simulink model "WMR_ROS_MATMPC_SIMULINK"  (R2022b)
settings: Solver=FixedStepAuto  StartTime=0.0  StopTime=20  FixedStep=0.001  RelTol=1e-3
values from neighbouring files (symbols this model uses):
  lb = 0    [Initialization_Simulink.m]
  lbu = -inf(nu,1)    [InitData.m]    (also in Initialization_Simulink.m = repmat(lbu,1,N))
  lbx = 0    [Initialization_Simulink.m]
  N = settings.N    [InitData.m]    (also in InitMemory.m; Initialization_Simulink.m = 160; Simulation.m = 10)
  para = repmat(para0,1,N+1)    [InitData.m]    (also in Initialization_Simulink.m)
  Ts = settings.Ts_st    [Initialization_Simulink.m]    (also in Simulation.m)
  ub = 0    [Initialization_Simulink.m]
  ubu = inf(nu,1)    [InitData.m]    (also in Initialization_Simulink.m = repmat(ubu,1,N))
  ubx = 0    [Initialization_Simulink.m]
  W = repmat([1 1 0.001 1 1 5 10]',1,N)    [Initialization_Simulink.m]
  WN = [100 100 0.001 10 10]'    [Initialization_Simulink.m]
  yref = 1    [run_experiment_gazebo.m]    (also in run_experiment_move_base.m; run_experiment_simulink.m = 2)
  z0 = 0    [Initialization_Simulink.m]
  zref = 2    [run_experiment_gazebo.m]    (also in run_experiment_move_base.m = 4; run_experiment_simulink.m = 4)
undefined symbols (not defined in the file or in its folder): Angular, Linear, opt, settings, X, X_SL_Info, Y, Y_SL_Info
libraries: robotlib x5, robotgazebolib x1, robotcorelib x1
settings Model: Creator=chen  LastModifiedBy=davidedl
settings SolverCC: AlgebraicLoopSolver=TrustRegion
settings DataIOCC: ReturnWorkspaceOutputs=off
settings OptimizationCC: EnhancedBackFolding=on  PassReuseOutputArgsAs=Individual arguments  ZeroExternalMemoryAtStartup=off  ZeroInternalMemoryAtStartup=off  MaxStackSize=64  OptimizeBlockOrder=speed  DifferentSizesBufferReuse=on  OptimizationCustomize=off  EfficientTunableParamExpr=on
settings DebuggingCC: ParameterTunabilityLossMsg=error  UnconnectedInputMsg=warning  UnconnectedOutputMsg=warning  UnconnectedLineMsg=warning  SFMachineParentedDataDiag=warning  ArithmeticOperatorsInVariantConditions=warning
settings HardwareCC: ProdBitPerPointer=32  ProdBitPerSizeT=32  ProdBitPerPtrDiffT=32  ProdLargestAtomicFloat=None  ProdIntDivRoundTo=Undefined  ProdEndianess=Unspecified  ProdWordSize=32  ProdHWDeviceType=Generic->Unspecified (assume 32-bit Generic)  UseEmbeddedCoderFeatures=off
settings ModelReferenceCC: EnableRefExpFcnMdlSchedulingChecks=on
settings SFSimCC: SimUseLocalCustomCode=off  MATLABDynamicMemAlloc=off  CustomCodeUndefinedFunction=UseInterfaceOnly
settings RTWCC: Description=Embedded Coder  SystemTargetFile=ert.tlc  HardwareBoard=Robot Operating System (ROS)  TLCOptions="-aInlineSetEventsForThisBaseRateFcn=TLC_FALSE -aSuppressMultiTaskScheduler=TLC_FALSE  -aRateBasedStepFcn=0"  TemplateMakefile=ert_default_tmf  RTWUseLocalCustomCode=off  Toolchain=Catkin  TargetLang=C++  CheckMdlBeforeBuild=Error
settings CodeAppCC: ForceParamTrailComments=on  IgnoreCustomStorageClasses=off  OperatorAnnotations=on  SimulinkDataObjDesc=on  SFDataObjDesc=on  InsertBlockDesc=on
settings ERTTargetCC: SupportNonInlinedSFcns=on

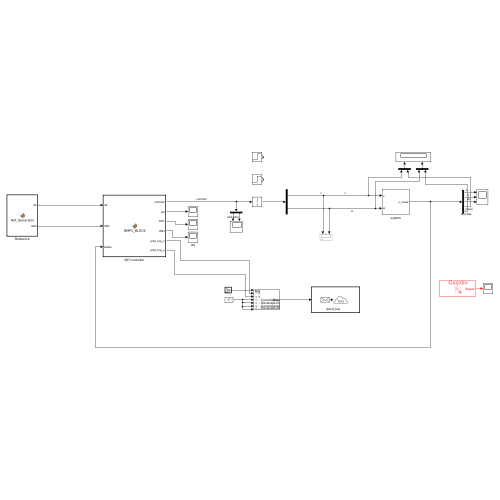
[thumbnail: Simulink's stored preview of the top-level diagram]
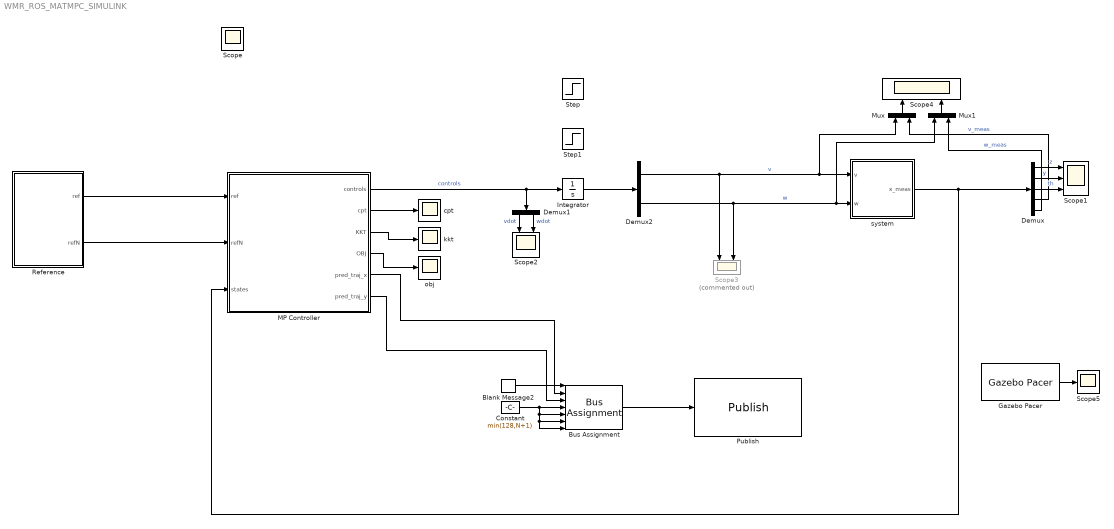
== system WMR_ROS_MATMPC_SIMULINK ==
  Blank Message2 : robotlib/Blank Message  messageClass=Message  entityType=wheelchair_iaslab_control/matArray  messageType=wheelchair_iaslab_control/matArray  SampleTime=-1  legacyBusStruct=off
  Bus Assignment : BusAssignment  AssignedSignals=X,Y,X_SL_Info.CurrentLength,X_SL_Info.ReceivedLength,Y_SL_Info.CurrentLength,Y_SL_Info.ReceivedLength
  Constant : Constant  Value=min(128,N+1)  OutDataTypeStr=uint32
  Demux : Demux  Outputs=5
  Demux1 : Demux  Outputs=2
  Demux2 : Demux  Outputs=2
  Gazebo Pacer : robotgazebolib/Gazebo Pacer  ResetBehavior=Reset Gazebo simulation time and scene  SampleTime=0.001
  Integrator : Integrator  InitialCondition=[0,0]
  MP Controller : MATLAB Function  TreatAsAtomicUnit=on  SystemSampleTime=Ts
  Mux : Mux  Inputs=2
  Mux1 : Mux  Inputs=2
  Publish : robotlib/Publish  topicSource=Specify your own  topic=/pred_traj  messageType=wheelchair_iaslab_control/matArray  legacyBusStruct=off  messageQueueLength=1
      settings: LibrarySourceBlock=roslib/ROS/Publish
  Reference : MATLAB Function  TreatAsAtomicUnit=on
  Scope1 : Scope  NumInputPorts=3
  Scope2 : Scope  NumInputPorts=2
  Scope3 : Scope  Commented=on  NumInputPorts=2
  Scope4 : Scope  NumInputPorts=2
  Scope5 : Scope
  Step : Step  Time=9  After=0  SampleTime=0
  Step1 : Step  Time=9  After=0  SampleTime=0
  cpt : Scope
  kkt : Scope
  obj : Scope
  system : Subsystem
  Scope : Scope
  wires:
  MP Controller/1(controls) -> Integrator/1, Demux1/1  "controls"
  MP Controller/2(cpt) -> cpt/1
  MP Controller/4(OBJ) -> obj/1
  MP Controller/3(KKT) -> kkt/1
  Reference/1(ref) -> MP Controller/1(ref)
  Reference/2(refN) -> MP Controller/2(refN)
  Integrator/1 -> Demux2/1
  Demux2/1 -> Scope3/1, Mux/1, system/1(v)  "v"
  Demux2/2 -> Mux1/1, system/2(w), Scope3/2  "w"
  Demux/3 -> Scope1/3  "th"
  Demux/1 -> Scope1/1  "z"
  Demux/2 -> Scope1/2  "y"
  Demux/5 -> Mux1/2  "w_meas"
  Demux/4 -> Mux/2  "v_meas"
  Demux1/1 -> Scope2/1  "vdot"
  Demux1/2 -> Scope2/2  "wdot"
  system/1(x_meas) -> MP Controller/3(states), Demux/1
  Mux/1 -> Scope4/1
  Mux1/1 -> Scope4/2
  Blank Message2/1 -> Bus Assignment/1
  Bus Assignment/1 -> Publish/1
  MP Controller/5(pred_traj_x) -> Bus Assignment/2
  MP Controller/6(pred_traj_y) -> Bus Assignment/3
  Gazebo Pacer/1 -> Scope5/1
  Constant/1 -> Bus Assignment/7, Bus Assignment/6, Bus Assignment/5, Bus Assignment/4

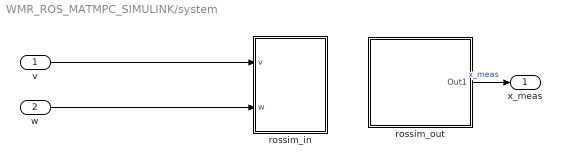
== system WMR_ROS_MATMPC_SIMULINK/system ==
  v : Inport
  w : Inport  Port=2
  rossim_in : Subsystem
  rossim_out : Subsystem
  x_meas : Outport
  wires:
  w/1 -> rossim_in/2(w)
  v/1 -> rossim_in/1(v)
  rossim_out/1(Out1) -> x_meas/1  "x_meas"

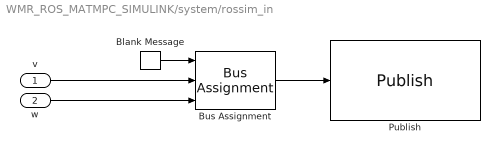
== system WMR_ROS_MATMPC_SIMULINK/system/rossim_in ==
  v : Inport
  w : Inport  Port=2
  Blank Message : robotlib/Blank Message  messageClass=Message  entityType=geometry_msgs/Twist  messageType=geometry_msgs/Twist  SampleTime=-1  legacyBusStruct=off
  Bus Assignment : BusAssignment  AssignedSignals=Linear.X,Angular.Z
  Publish : robotlib/Publish  topicSource=Specify your own  topic=/wcias_controller/cmd_vel  messageType=geometry_msgs/Twist  legacyBusStruct=off  messageQueueLength=1
      settings: LibrarySourceBlock=roslib/ROS/Publish
  wires:
  Blank Message/1 -> Bus Assignment/1
  Bus Assignment/1 -> Publish/1
  w/1 -> Bus Assignment/3
  v/1 -> Bus Assignment/2

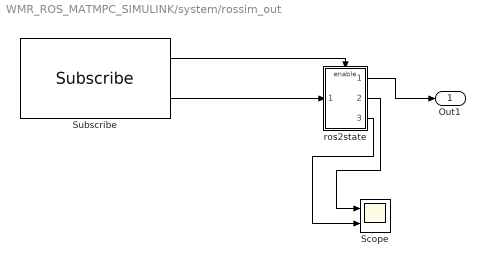
== system WMR_ROS_MATMPC_SIMULINK/system/rossim_out ==
  Scope : Scope  NumInputPorts=2
  Subscribe : robotlib/Subscribe  topicSource=Specify your own  topic=/wcias_controller/odom  messageType=nav_msgs/Odometry  SampleTime=0.001  legacyBusStruct=off  messageQueueLength=1
      settings: LibrarySourceBlock=roslib/ROS/Subscribe
  ros2state : Subsystem
  Out1 : Outport
  wires:
  Subscribe/1 -> ros2state/Enable
  Subscribe/2 -> ros2state/1(In1)
  ros2state/1(Out1) -> Out1/1
  ros2state/2(Out2) -> Scope/1
  ros2state/3(Out3) -> Scope/2

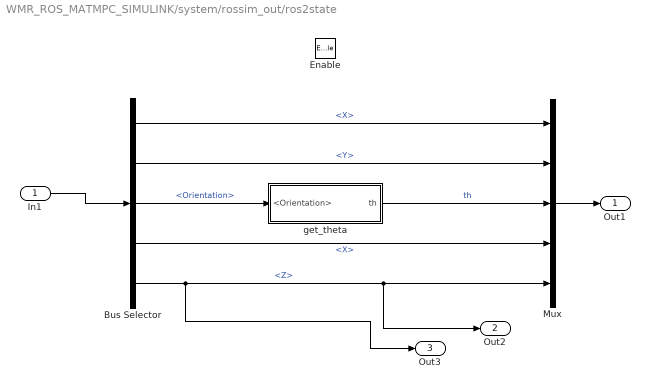
== system WMR_ROS_MATMPC_SIMULINK/system/rossim_out/ros2state ==
  In1 : Inport
  Enable : EnablePort  StatesWhenEnabling=reset
  Bus Selector : BusSelector  DialogController=Simulink.DDGSource_BusSelector  OutputSignals=Pose.Pose.Position.X,Pose.Pose.Position.Y,Pose.Pose.Orientation,Twist.Twist.Linear.X,Twist.Twist.Angular.Z
  Mux : Mux  Inputs=5
  get_theta : Subsystem
  Out1 : Outport
  Out2 : Outport  Port=2
  Out3 : Outport  Port=3
  wires:
  Bus Selector/5 -> Mux/5, Out2/1, Out3/1  "<Z>"
  Bus Selector/1 -> Mux/1  "<X>"
  In1/1 -> Bus Selector/1
  get_theta/1(th) -> Mux/3  "th"
  Bus Selector/2 -> Mux/2  "<Y>"
  Bus Selector/3 -> get_theta/1(<Orientation>)  "<Orientation>"
  Bus Selector/4 -> Mux/4  "<X>"
  Mux/1 -> Out1/1

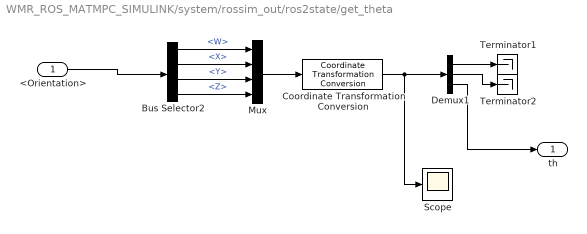
== system WMR_ROS_MATMPC_SIMULINK/system/rossim_out/ros2state/get_theta ==
  <Orientation> : Inport
  Bus Selector2 : BusSelector  DialogController=Simulink.DDGSource_BusSelector  OutputSignals=W,X,Y,Z
  Coordinate Transformation Conversion : robotcorelib/Coordinate Transformation Conversion  InputRepresentation=Quaternion  InputEulerSequence=ZYX  ShowTrVecInputPort=on  OutputRepresentation=Euler Angles  OutputEulerSequence=XYZ  ShowTrVecOutputPort=on  SimulateUsing=Interpreted execution
      settings: LibrarySourceBlock=roslib/Utilities/Coordinate Transformation Conversion
  Demux1 : Demux  Outputs=3
  Mux : Mux
  Scope : Scope
  Terminator1 : Terminator
  Terminator2 : Terminator
  th : Outport
  wires:
  Bus Selector2/3 -> Mux/3  "<Y>"
  Demux1/1 -> Terminator1/1
  Bus Selector2/4 -> Mux/4  "<Z>"
  Bus Selector2/1 -> Mux/1  "<W>"
  Coordinate Transformation Conversion/1 -> Scope/1, Demux1/1
  <Orientation>/1 -> Bus Selector2/1
  Demux1/2 -> Terminator2/1
  Bus Selector2/2 -> Mux/2  "<X>"
  Mux/1 -> Coordinate Transformation Conversion/1
  Demux1/3 -> th/1

== matlab function WMR_ROS_MATMPC_SIMULINK/Reference ==
  data: ref output; settings parameter; refN output; zref parameter; yref parameter
function [ref,refN] = Ref_Generator(settings, zref, yref)

    ref = repmat([zref,yref,0,0,0,0,0]',1,settings.N);
    refN = [zref,yref,0,0,0]';

end

== matlab function WMR_ROS_MATMPC_SIMULINK/MP Controller ==
  settings: updateMethod=DISCRETE  sampleTime=1/50
  data: settings parameter; opt parameter; lb parameter; ub parameter; lbx parameter; ubx parameter; lbu parameter; ubu parameter; W parameter; WN parameter; para parameter; ref input size=[ny N]; refN input size=nyN; z0 parameter; states input size=nx; controls output size=nu; cpt output size=1; KKT output; OBJ output; pred_traj_x output; pred_traj_y output; N parameter
function [controls, cpt, KKT, OBJ,pred_traj_x,pred_traj_y]  = NMPC_BLOCK(settings, opt, lb, ub, lbx, ubx, lbu, ubu, W, WN, para, ref, refN, z0, states,N)

%% everything should have a fixed size
coder.extrinsic('mpc_nmpcsolver_simulink');  
coder.extrinsic('InitData');  
coder.extrinsic('InitMemory');  
coder.extrinsic('evalin');
coder.extrinsic('assignin');

%%

persistent x u z lambda mu mu_x mu_u;
persistent input mem;

if isempty(input)  
    
    nx = settings.nx;        % No. of differential states
    nu = settings.nu;        % No. of controls
    nz = settings.nz;        % No. of algebraic states
    ny = settings.ny;        % No. of outputs (references)    
    nyN= settings.nyN;       % No. of outputs at terminal stage 
    np = settings.np;        % No. of parameters (on-line data)
    nc = settings.nc;        % No. of constraints
    ncN = settings.ncN;      % No. of constraints at terminal stage
    nbu = settings.nbu;      % No. of control bounds
    nbx = settings.nbx;      % No. of state bounds
    nbu_idx = settings.nbu_idx; % Index of control bounds
    nbx_idx = settings.nbx_idx; % Index of state bounds
    N = settings.N;
    N2 = settings.N2;
    r = settings.r;
        
    input.x0=states;
    
    x=repmat(states,1,N+1);
    input.x=x;
    
    u=zeros(nu,N);
    input.u=u;
    
    z=repmat(z0,1,N);
    input.z=z;
    
    lambda = zeros(nx,N+1);
    input.lambda= lambda;
    
    if N*nc+ncN > 0
        mu = zeros(N*nc+ncN,1);
    else
        mu = 0;
    end
    input.mu= mu;
    
    mu_u = zeros(N*nu,1);
    input.mu_u= mu_u;
    
    if N*nbx > 0
        mu_x = zeros(N*nbx,1);
    else
        mu_x = 0;
    end
    input.mu_x = mu_x;
    
    input.W=W;
    input.WN=WN;
    input.od = para;
    
    input.lb = lb;
    input.ub = ub;
    input.lbx = lbx;
    input.ubx = ubx;
    input.lbu = lbu;
    input.ubu = ubu;
      
    input.y = ref;
    input.yN = refN;
    
    mem = InitMemory(settings, opt, input);
        
else

    input.x=x; 
    input.u=u;
    input.z=z;
    input.lambda=lambda;   
    input.mu=mu;
    input.mu_x=mu_x;
    input.mu_u=mu_u;
    
end

%%
cpt = 0;
KKT = 0;
OBJ = 0;
input.x0 = states;

%%DAVIDE
pred_traj_x = zeros(128,1);
pred_traj_y = zeros(128,1);

pred_traj_x(1:min(N+1,128)) = input.x(1,1:min(128,N+1))';
pred_traj_y(1:min(N+1,128)) = input.x(2,1:min(128,N+1))';

[input,mem,cpt,KKT,OBJ] = mpc_nmpcsolver_simulink(input, settings, mem, opt);
controls = input.u(:,1);

%% shifting
switch opt.shifting
    case 'yes'
        x=[input.x(:,2:end),input.x(:,end)];  
        u=[input.u(:,2:end),input.u(:,end)]; 
        z=[input.z(:,2:end),input.z(:,end)]; 
        lambda=[input.lambda(:,2:end),input.lambda(:,end)];
        if (settings.N*settings.nc+settings.ncN) >0
            mu(1:end-settings.ncN+1)=input.mu(settings.nc+1:settings.N*settings.nc+settings.ncN,1);
            mu(settings.N*settings.nc+1:end)=input.mu(settings.N*settings.nc+settings.ncN-settings.nc+1:settings.N*settings.nc+settings.ncN,1);
        else
            mu=0;
        end
        mu_x=[input.mu_x(2:end,1);input.mu_x(end,1)];
        mu_u=[input.mu_u(2:end,1);input.mu_u(end,1)];
   case 'no'
        x=input.x;
        u=input.u;
        z=input.z;
        lambda=input.lambda;
        mu=input.mu;
        mu_x=input.mu_x;
        mu_u=input.mu_u;
end

return
